simulink subsystem "Odemetria"  (R2023b)
settings: Solver=VariableStepAuto  StartTime=0.0  StopTime=10.0  RelTol=1e-3
settings Model: Creator=adria  LastModifiedBy=adria

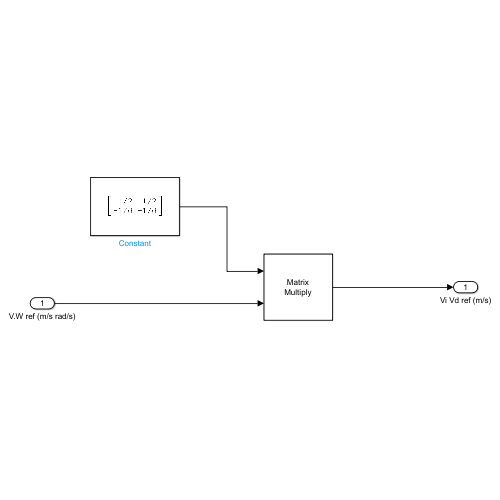
[thumbnail: Simulink's stored preview of the top-level diagram]
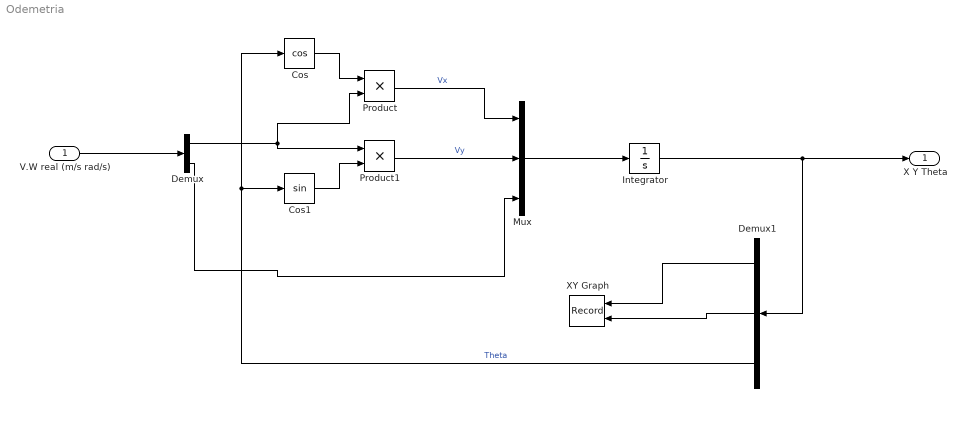
== system Odemetria ==
  V.W real (m/s rad/s) : Inport  OutDataTypeStr=double  PortDimensions=2
  Cos : Trigonometry  Operator=cos
  Cos1 : Trigonometry
  Demux : Demux  Outputs=2
  Demux1 : Demux  Outputs=3
  Integrator : Integrator
  Mux : Mux  Inputs=3
  Product : Product
  Product1 : Product
  XY Graph : Record  FileSettingsInternal="{\"entries\":[{\"content\":{\"excelSettings\":{\"content\":{},\"type\":\"Streamout.ExcelSettings\"}},\"type\":\"Streamout.FileSettingStorage\",\"uuid\":\"\"}],\"packageUris\":[\"http:\\/\\/schema.mathworks.com\\/mf0\\/streamout_blocks\\/R2020a\"],\"version\":\"1.0\"}"  Layout=[1 1]  SignalsInternal="{\"entries\":[{\"content\":{\"signals\":[{\"content\":{\"blockPath\":[],\"dimensions\":[1],\"domain\":\"\",\"lineColor\":\"#a2142f\",\"plots\":[1],\"port\":1,\"signalID\":4787,\"signalName\":\"XY Graph:1\"},\"type\":\"RecordBlkView.Signal\",\"uuid\":\"\"},{\"content\":{\"blockPath\":[],\"dimensions\":[1],\"domain\":\"\",\"lineColor\":\"#139fff\",\"plots\":[1],\"port\":2,\"signalID\":4790,\"signalName\":\"XY Graph:2\"},\"type\":\"RecordBlkView.Signal\",\"uuid\":\"\"}]},\"type\":\"RecordBlkView.InputSignals\",\"uuid\":\"\"}],\"packageUris\":[\"http:\\/\\/schema.mathworks.com\\/mf0\\/streamout_blocks\\/R2020a\"],\"version\":\"1.0\"}"  VisualizationBindings="{\"xyplotplugin\":{\"info\":[{\"series\":[{\"bindingParametersList\":[{\"parameter\":\"X-Axis\",\"signalID\":4787,\"signalName\":\"XY Graph:1\"},{\"parameter\":\"Y-Axis\",\"signalID\":4790,\"signalName\":\"XY Graph:2\"}],\"seriesID\":434}],\"subplotID\":1}]}}"  CompatibilityTag=XY
  X Y Theta : Outport
  wires:
  V.W real (m/s rad/s)/1 -> Demux/1
  Product/1 -> Mux/1  "Vx"
  Product1/1 -> Mux/2  "Vy"
  Integrator/1 -> X Y Theta/1, Demux1/1
  Demux/2 -> Mux/3
  Demux/1 -> Product1/1, Product/2
  Mux/1 -> Integrator/1
  Cos/1 -> Product/1
  Demux1/1 -> XY Graph/1
  Demux1/2 -> XY Graph/2
  Demux1/3 -> Cos1/1, Cos/1  "Theta"
  Cos1/1 -> Product1/2
